simulink model "schema_arthur"  (R2021a)
settings: Solver=VariableStepAuto  StartTime=0.0  StopTime=10.0  RelTol=1e-3
values from neighbouring files (symbols this model uses):
  S = tf(S,1,Te)/z^2    [main_arthur.m]
libraries: cstblocks x31
settings Model: Creator=Usuario  LastModifiedBy=Arthur
settings SolverCC: AlgebraicLoopSolver=TrustRegion
settings DataIOCC: Refine=4
settings DebuggingCC: SFMachineParentedDataDiag=warning

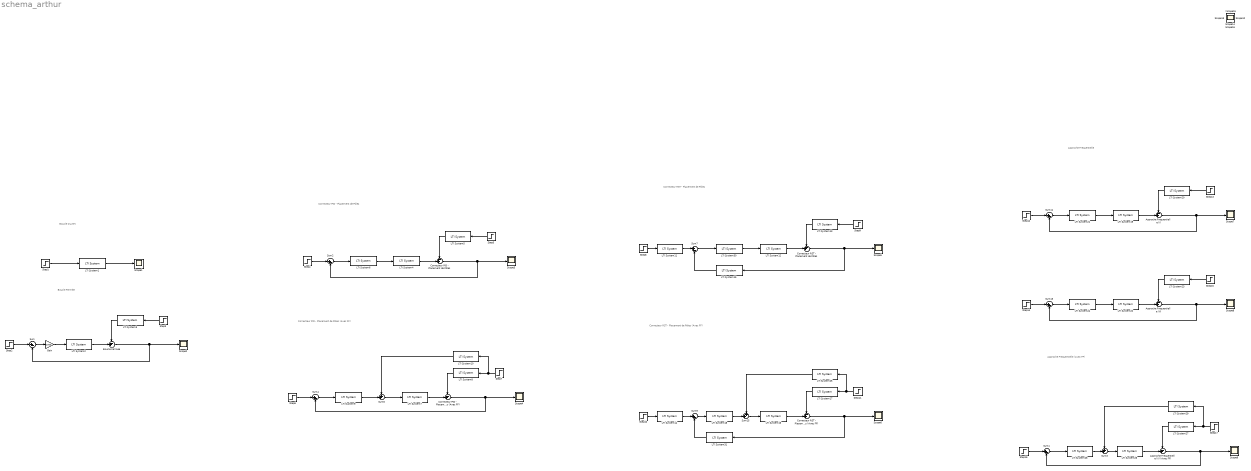
== system schema_arthur ==
  note: Boucle Ouvert
  note: Boucle Fermée
  note: Correcteur PID - Placement de Pôles
  note: Correcteur PID - Placement de Pôles (Avec FF)
  note: Correcteur RST - Placement de Pôles
  note: Approche Frequentielle
  note: Correcteur RST - Placement de Pôles (Avec FF)
  note: Approche Frequentielle (Avec FF)
  Approche Frequentielle (I) : Sum  Inputs=-+|
  Approche Frequentielle (II) : Sum  Inputs=-+|
  Approche Frequentielle (II) (Avec FF) : Sum  Inputs=-+|
  Boucle Fermée : Sum  Inputs=-+|
  Correcteur PID - Placement de Pôles : Sum  Inputs=-+|
  Correcteur PID - Placement de Pôles (Avec FF) : Sum  Inputs=-+|
  Correcteur RST - Placement de Pôles : Sum  Inputs=-+|
  Correcteur RST - Placement de Pôles (Avec FF) : Sum  Inputs=-+|
  Gain : Gain  Gain=1000
  LTI System{1..2,4,7,12,16,19,22,26} (9 alike) : cstblocks/LTI System  sys=TF2  IC=[]
  LTI System10 : cstblocks/LTI System  sys=FF  IC=[]
  LTI System11 : cstblocks/LTI System  sys=T  IC=[]
  LTI System{3,5,8,13,17,20,23,27} (8 alike) : cstblocks/LTI System  sys=TF3  IC=[]
  LTI System14 : cstblocks/LTI System  sys=T  IC=[]
  LTI System15 : cstblocks/LTI System  sys=R  IC=[]
  LTI System18 : cstblocks/LTI System  sys=1/S  IC=[]
  LTI System21 : cstblocks/LTI System  sys=KPIDI  IC=[]
  LTI System24 : cstblocks/LTI System  sys=KPIDII  IC=[]
  LTI System25 : cstblocks/LTI System  sys=FF  IC=[]
  LTI System28 : cstblocks/LTI System  sys=KPIDII  IC=[]
  LTI System29 : cstblocks/LTI System  sys=FF  IC=[]
  LTI System30 : cstblocks/LTI System  sys=1/S  IC=[]
  LTI System31 : cstblocks/LTI System  sys=R  IC=[]
  LTI System6 : cstblocks/LTI System  sys=Kpid  IC=[]
  LTI System9 : cstblocks/LTI System  sys=Kpid  IC=[]
  Scope{,1..16} (17 alike) : Scope
  Step{1..2,4,6,8,10,12,14,16} (9 alike) : Step  SampleTime=0
  Step{3,5,7,9,11,13,15,17} (8 alike) : Step  Time=5  SampleTime=0
  Sum{,1..2,4,7,9,11,13} (8 alike) : Sum  Inputs=|+-
  Sum15 : Sum  Inputs=++|
  Sum3 : Sum  Inputs=++|
  Sum6 : Sum  Inputs=++|
  wires:
  Step1/1 -> LTI System1/1
  LTI System1/1 -> Scope1/1
  Step2/1 -> Sum/1
  LTI System2/1 -> Boucle Fermée/2
  Sum/1 -> Gain/1
  Gain/1 -> LTI System2/1
  LTI System3/1 -> Boucle Fermée/1
  Step3/1 -> LTI System3/1
  Boucle Fermée/1 -> Sum/2, Scope2/1
  LTI System4/1 -> Correcteur PID - Placement de Pôles/2
  Sum2/1 -> LTI System6/1
  Step5/1 -> LTI System5/1
  LTI System5/1 -> Correcteur PID - Placement de Pôles/1
  Correcteur PID - Placement de Pôles/1 -> Sum2/2, Scope3/1
  Step4/1 -> Sum2/1
  LTI System6/1 -> LTI System4/1
  Sum4/1 -> LTI System9/1
  LTI System9/1 -> Sum6/2
  Step6/1 -> Sum4/1
  Step7/1 -> LTI System10/1, LTI System8/1
  LTI System8/1 -> Correcteur PID - Placement de Pôles (Avec FF)/1
  Correcteur PID - Placement de Pôles (Avec FF)/1 -> Sum4/2, Scope4/1
  LTI System7/1 -> Correcteur PID - Placement de Pôles (Avec FF)/2
  Sum6/1 -> LTI System7/1
  LTI System10/1 -> Sum6/1
  LTI System30/1 -> LTI System12/1
  LTI System12/1 -> Correcteur RST - Placement de Pôles/2
  Correcteur RST - Placement de Pôles/1 -> LTI System15/1, Scope5/1
  Step8/1 -> LTI System11/1
  LTI System13/1 -> Correcteur RST - Placement de Pôles/1
  Step9/1 -> LTI System13/1
  Sum7/1 -> LTI System30/1
  LTI System11/1 -> Sum7/1
  LTI System15/1 -> Sum7/2
  Sum11/1 -> LTI System21/1
  LTI System21/1 -> LTI System19/1
  Step12/1 -> Sum11/1
  Step13/1 -> LTI System20/1
  LTI System20/1 -> Approche Frequentielle (I)/1
  Approche Frequentielle (I)/1 -> Sum11/2, Scope7/1
  LTI System19/1 -> Approche Frequentielle (I)/2
  Approche Frequentielle (II)/1 -> Sum13/2, Scope8/1
  LTI System23/1 -> Approche Frequentielle (II)/1
  LTI System22/1 -> Approche Frequentielle (II)/2
  Sum13/1 -> LTI System24/1
  Step15/1 -> LTI System23/1
  Step14/1 -> Sum13/1
  LTI System24/1 -> LTI System22/1
  Sum9/1 -> LTI System18/1
  LTI System31/1 -> Sum9/2
  LTI System17/1 -> Correcteur RST - Placement de Pôles (Avec FF)/1
  Step10/1 -> LTI System14/1
  LTI System16/1 -> Correcteur RST - Placement de Pôles (Avec FF)/2
  Correcteur RST - Placement de Pôles (Avec FF)/1 -> LTI System31/1, Scope6/1
  LTI System18/1 -> Sum15/2
  LTI System14/1 -> Sum9/1
  LTI System25/1 -> Sum15/1
  Step11/1 -> LTI System25/1, LTI System17/1
  Sum15/1 -> LTI System16/1
  Sum1/1 -> LTI System28/1
  Step16/1 -> Sum1/1
  LTI System26/1 -> Approche Frequentielle (II) (Avec FF)/2
  LTI System28/1 -> Sum3/2
  LTI System27/1 -> Approche Frequentielle (II) (Avec FF)/1
  Approche Frequentielle (II) (Avec FF)/1 -> Sum1/2, Scope9/1
  Step17/1 -> LTI System29/1, LTI System27/1
  LTI System29/1 -> Sum3/1
  Sum3/1 -> LTI System26/1
